simulink model "dwwwdq"  (R2020b)
settings: Solver=VariableStepDiscrete  StartTime=0.0  StopTime=0.3  MaxStep=1e-5  RelTol=1e-3
settings Model: Creator=seojoon  LastModifiedBy=seojoon

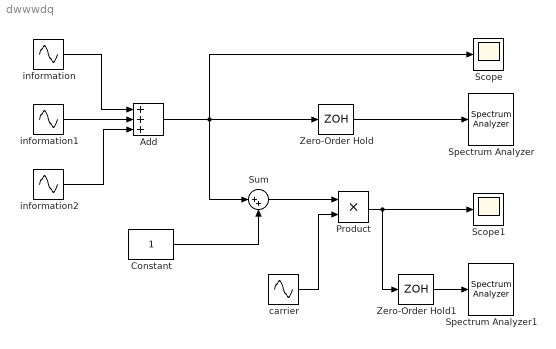
== system dwwwdq ==
  Add : Sum  Inputs=+++
  Constant : Constant
  Product : Product
  Scope : Scope
  Scope1 : Scope
  Spectrum Analyzer : SpectrumAnalyzer
  Spectrum Analyzer1 : SpectrumAnalyzer
  Sum : Sum  Inputs=|++
  Zero-Order Hold : ZeroOrderHold  SampleTime=0.3/4096
  Zero-Order Hold1 : ZeroOrderHold  SampleTime=0.3/4096
  carrier : Sin  Frequency=2*pi*3000  Phase=pi/2  SampleTime=0
  information : Sin  Amplitude=0.7  Frequency=2*pi*40  SampleTime=0
  information1 : Sin  Frequency=2*pi*120  Phase=pi/2  SampleTime=0
  information2 : Sin  Amplitude=-0.6  Frequency=2*pi*160  Phase=pi/2  SampleTime=0
  wires:
  information/1 -> Add/1
  Constant/1 -> Sum/2
  Sum/1 -> Product/1
  carrier/1 -> Product/2
  Product/1 -> Zero-Order Hold1/1, Scope1/1
  Zero-Order Hold/1 -> Spectrum Analyzer/1
  Zero-Order Hold1/1 -> Spectrum Analyzer1/1
  information1/1 -> Add/2
  information2/1 -> Add/3
  Add/1 -> Sum/1, Scope/1, Zero-Order Hold/1
